simulink model "P_decouple_cascade_rov"  (Simulink 6.0)
settings: Solver=ode45  StartTime=0.0  StopTime=650  RelTol=1e-3
undefined symbols (not defined in the file): B, DQ, DQL, I, m, M, Ma, MaL, MaU, rg, sigbuilder_block, T, W, xb, xg, Xudot, yb, yg, Yvdot, zb, zg, Zwdot
libraries: simulink_extras x27, simulink x20
(part 3 of 5)

== system P_decouple_cascade_rov/outer-loop  controller/PI sine +nonlinear /Subsystem ==
  xe : Inport  Port=1  LatchInput=off
  ye : Inport  Port=2  LatchInput=off
  Divide : Product  Inputs=**/  OutScaling=2^-10
  Divide1 : Product  Inputs=**  OutScaling=2^-10
  Divide2 : Product  Inputs=***  OutScaling=2^-10
  Gain : Gain  Gain=-1
  Sine Wave : Sin  Frequency=5  Phase=pi/2  SampleTime=0
  Subtract : Sum  Inputs=+++  OutScaling=2^-10
  Subtract1 : Sum  OutScaling=2^-10
  Trigonometric Function : Trigonometry  Operator=asin
  lamda 0 : Constant  Value=0.1
  lamda 1 : Constant  Value=0.3
  lamda 2 : Constant  Value=0.5
  lamda0^2 : Math  Operator=square  SaturateOnIntegerOverflow=on
  ud : Constant  Value=0.5
  xe^2 : Math  Operator=square  SaturateOnIntegerOverflow=on
  ye^2 : Math  Operator=square  SaturateOnIntegerOverflow=on
  yaw_angle : Outport
  wires:
  lamda 0/1 -> lamda0^2/1
  lamda0^2/1 -> Subtract/1
  xe^2/1 -> Subtract/2
  ye^2/1 -> Subtract/3
  Subtract/1 -> Divide/3
  lamda 1/1 -> Divide1/1, Divide2/1
  ud/1 -> Divide1/2
  Divide1/1 -> Subtract1/1
  Divide2/1 -> Subtract1/2
  lamda 2/1 -> Divide2/2
  Sine Wave/1 -> Divide2/3
  Trigonometric Function/1 -> Gain/1
  Subtract1/1 -> Divide/1
  Divide/1 -> Trigonometric Function/1
  xe/1 -> xe^2/1
  ye/1 -> ye^2/1, Divide/2
  Gain/1 -> yaw_angle/1

== system P_decouple_cascade_rov/outer-loop  controller/outer-P decouple /inner-PI ==
  PI : Inport  Port=1  LatchInput=off
  Demux1 : Demux  Outputs=6
  Mux2 : Mux  Inputs=6
  P Controller2 : simulink_extras/Additional Linear/PID Controller  P=1  I=0  D=0
  P Controller4 : simulink_extras/Additional Linear/PID Controller  P=1  I=0  D=0
  PController1 : simulink_extras/Additional Linear/PID Controller  P=1  I=0  D=0
  PI Controller3 : simulink_extras/Additional Linear/PID Controller  P=1  I=0  D=0
  " " : Outport
  wires:
  PI Controller3/1 -> Mux2/3
  PController1/1 -> Mux2/1
  P Controller2/1 -> Mux2/2
  Demux1/1 -> PController1/1
  Demux1/2 -> P Controller2/1
  Demux1/3 -> PI Controller3/1
  Demux1/6 -> P Controller4/1
  P Controller4/1 -> Mux2/6
  PI/1 -> Demux1/1
  Mux2/1 -> " "/1

== system P_decouple_cascade_rov/outer-loop  controller/outer-sliding decouple/Subsystem ==
  xe : Inport  Port=1  LatchInput=off
  ye : Inport  Port=2  LatchInput=off
  Divide : Product  Inputs=**/  OutScaling=2^-10
  Divide1 : Product  Inputs=**  OutScaling=2^-10
  Divide2 : Product  Inputs=***  OutScaling=2^-10
  Gain : Gain  Gain=-1
  Sine Wave : Sin  Frequency=5  Phase=pi/2  SampleTime=0
  Subtract : Sum  Inputs=+++  OutScaling=2^-10
  Subtract1 : Sum  OutScaling=2^-10
  Trigonometric Function : Trigonometry  Operator=asin
  lamda 0 : Constant  Value=0.1
  lamda 1 : Constant  Value=0.3
  lamda 2 : Constant  Value=0.5
  lamda0^2 : Math  Operator=square  SaturateOnIntegerOverflow=on
  ud : Constant  Value=0.5
  xe^2 : Math  Operator=square  SaturateOnIntegerOverflow=on
  ye^2 : Math  Operator=square  SaturateOnIntegerOverflow=on
  yaw_angle : Outport
  wires:
  lamda 0/1 -> lamda0^2/1
  lamda0^2/1 -> Subtract/1
  xe^2/1 -> Subtract/2
  ye^2/1 -> Subtract/3
  Subtract/1 -> Divide/3
  lamda 1/1 -> Divide1/1, Divide2/1
  ud/1 -> Divide1/2
  Divide1/1 -> Subtract1/1
  Divide2/1 -> Subtract1/2
  lamda 2/1 -> Divide2/2
  Sine Wave/1 -> Divide2/3
  Trigonometric Function/1 -> Gain/1
  Subtract1/1 -> Divide/1
  Divide/1 -> Trigonometric Function/1
  xe/1 -> xe^2/1
  ye/1 -> ye^2/1, Divide/2
  Gain/1 -> yaw_angle/1

== system P_decouple_cascade_rov/pipeline  tracking planner  /decoupled input/x25, y=0, z=50 yaw=1.57 ==
  Mux : Mux  Inputs=6
  Start : Constant  Value=15
  Start1 : Constant  Value=25
  Start2 : Constant  Value=1.57
  6 : Outport
  wires:
  Start1/1 -> Mux/1
  Mux/1 -> 6/1
  Start2/1 -> Mux/6
  Start/1 -> Mux/3

== system P_decouple_cascade_rov/pipeline  tracking planner  /decoupled input/x=0,y=0, z=0 yaw=0   ==
  Mux : Mux  Inputs=6
  Start : Constant  Value=0
  Start1 : Constant  Value=0
  8 : Outport
  wires:
  Mux/1 -> 8/1
  Start1/1 -> Mux/1
  Start/1 -> Mux/3, Mux/2, Mux/6

== system P_decouple_cascade_rov/pipeline  tracking planner  /decoupled input/x=15,y=0, z=45 yaw=0  ==
  Mux : Mux  Inputs=6
  Start1 : Constant  Value=15
  Start2 : Constant  Value=10
  Start3 : Constant  Value=0
  Start4 : Constant  Value=0
  3 : Outport
  wires:
  Mux/1 -> 3/1
  Start1/1 -> Mux/1
  Start2/1 -> Mux/3
  Start3/1 -> Mux/6
  Start4/1 -> Mux/2

== system P_decouple_cascade_rov/pipeline  tracking planner  /decoupled input/x=25, z=45 yaw=0 ==
  Mux : Mux  Inputs=6
  Start : Constant  Value=10
  Start1 : Constant  Value=25
  Start2 : Constant  Value=0
  4 : Outport
  wires:
  Mux/1 -> 4/1
  Start1/1 -> Mux/1
  Start/1 -> Mux/3
  Start2/1 -> Mux/6

== system P_decouple_cascade_rov/pipeline  tracking planner  /decoupled input/x=25,y=0, z=50 yaw=0 ==
  Mux : Mux  Inputs=6
  Start : Constant  Value=0
  Start1 : Constant  Value=25
  Start2 : Constant  Value=15
  5 : Outport
  wires:
  Start1/1 -> Mux/1
  Mux/1 -> 5/1
  Start/1 -> Mux/6
  Start2/1 -> Mux/3

== system P_decouple_cascade_rov/pipeline  tracking planner  /decoupled input/x=25,y=40, z=50 yaw=0 ==
  Mux : Mux  Inputs=6
  Start : Constant  Value=0
  Start1 : Constant  Value=25
  Start2 : Constant  Value=15
  Start3 : Constant  Value=15
  7 : Outport
  wires:
  Start1/1 -> Mux/1
  Mux/1 -> 7/1
  Start/1 -> Mux/6
  Start2/1 -> Mux/2
  Start3/1 -> Mux/3

== system P_decouple_cascade_rov/pipeline  tracking planner  /decoupled input/x=y=0, z=-50 yaw=0   ==
  Mux : Mux  Inputs=6
  Start : Constant  Value=15
  Start1 : Constant  Value=0
  Start2 : Constant  Value=0
  "1 " : Outport
  wires:
  Mux/1 -> "1 "/1
  Start1/1 -> Mux/1, Mux/2
  Start/1 -> Mux/3
  Start2/1 -> Mux/6

== system P_decouple_cascade_rov/pipeline  tracking planner  /decoupled input/x=y=15, z=50 yaw=0  ==
  Mux : Mux  Inputs=6
  Start : Constant  Value=0
  Start1 : Constant  Value=15
  Start2 : Constant  Value=15
  2 : Outport
  wires:
  Mux/1 -> 2/1
  Start1/1 -> Mux/1
  Start2/1 -> Mux/3
  Start/1 -> Mux/6

== system P_decouple_cascade_rov/(Observer/Euler  Transformation1/Transformation matrix R/Row1 of T ==
  angular body  velocity : Inport  Port=1  LatchInput=off
  angular position : Inport  Port=2  LatchInput=off
  1 : Fcn  Expr=1
  Dot Product1 : simulink/Math Operations/Dot Product  InputSameDT=on  OutDataType=sfix(16)  OutScaling=2^-10  DoSatur=off
  Mux1 : Mux  Inputs=3
  cX.tY : Fcn  Expr=cos(u[1])*tan(u[2])
  sX.tY : Fcn  Expr=sin(u[1])*tan(u[2])
  angular earth velocity (row 1) : Outport
  wires:
  Dot Product1/1 -> angular earth velocity (row 1)/1
  angular body  velocity/1 -> Dot Product1/2
  Mux1/1 -> Dot Product1/1
  cX.tY/1 -> Mux1/3
  sX.tY/1 -> Mux1/2
  1/1 -> Mux1/1
  angular position/1 -> cX.tY/1, sX.tY/1, 1/1

== system P_decouple_cascade_rov/(Observer/Euler  Transformation1/Transformation matrix R/Row2 of T ==
  "angular body velocity " : Inport  Port=1  LatchInput=off
  angular position : Inport  Port=2  LatchInput=off
  -sX : Fcn  Expr=-sin(u[1])
  0 : Fcn  Expr=0
  Dot Product1 : simulink/Math Operations/Dot Product  InputSameDT=on  OutDataType=sfix(16)  OutScaling=2^-10  DoSatur=off
  Mux1 : Mux  Inputs=3
  cX : Fcn  Expr=cos(u[1])
  angular earth velocity (row 2) : Outport
  wires:
  Dot Product1/1 -> angular earth velocity (row 2)/1
  "angular body velocity "/1 -> Dot Product1/2
  Mux1/1 -> Dot Product1/1
  -sX/1 -> Mux1/3
  cX/1 -> Mux1/2
  0/1 -> Mux1/1
  angular position/1 -> -sX/1, cX/1, 0/1

== system P_decouple_cascade_rov/(Observer/Euler  Transformation1/Transformation matrix R/Row3 of T ==
  "angular body velocity " : Inport  Port=1  LatchInput=off
  angular position : Inport  Port=2  LatchInput=off
  1 : Fcn  Expr=0
  Dot Product1 : simulink/Math Operations/Dot Product  InputSameDT=on  OutDataType=sfix(16)  OutScaling=2^-10  DoSatur=off
  Mux1 : Mux  Inputs=3
  cX/cY : Fcn  Expr=cos(u[1])/cos(u[2])
  sX/cY : Fcn  Expr=sin(u[1])/cos(u[2])
  angular earth velocity (row 3) : Outport
  wires:
  Dot Product1/1 -> angular earth velocity (row 3)/1
  "angular body velocity "/1 -> Dot Product1/2
  Mux1/1 -> Dot Product1/1
  cX/cY/1 -> Mux1/3
  sX/cY/1 -> Mux1/2
  1/1 -> Mux1/1
  angular position/1 -> cX/cY/1, sX/cY/1, 1/1

== system P_decouple_cascade_rov/(Observer/Euler  Transformation1/Transformation matrix T/Row1 of R ==
  translational body velocity : Inport  Port=1  LatchInput=off
  angular position : Inport  Port=2  LatchInput=off
  -sZ.cX+cZ.sY.sX : Fcn  Expr=-sin(u[3])*cos(u[1]) + cos(u[3])*sin(u[2])*sin(u[1])
  Dot Product : simulink/Math Operations/Dot Product  InputSameDT=on  OutDataType=sfix(16)  OutScaling=2^-10  DoSatur=off
  Mux : Mux  Inputs=3
  cY.cZ : Fcn  Expr=cos(u[3]) * cos(u[2])
  sZ.sX+cZ.cX.sY : Fcn  Expr=sin(u[3])*sin(u[1]) + cos(u[3])*cos(u[1])*sin(u[2])
  translational earth velocity (row 1) : Outport
  wires:
  Dot Product/1 -> translational earth velocity (row 1)/1
  translational body velocity/1 -> Dot Product/2
  Mux/1 -> Dot Product/1
  sZ.sX+cZ.cX.sY/1 -> Mux/3
  -sZ.cX+cZ.sY.sX/1 -> Mux/2
  cY.cZ/1 -> Mux/1
  angular position/1 -> sZ.sX+cZ.cX.sY/1, -sZ.cX+cZ.sY.sX/1, cY.cZ/1

== system P_decouple_cascade_rov/(Observer/Euler  Transformation1/Transformation matrix T/Row2 of R ==
  translational body velocity : Inport  Port=1  LatchInput=off
  angular position : Inport  Port=2  LatchInput=off
  -cZ.sX+sY.sZ.cX : Fcn  Expr=-cos(u[3])*sin(u[1]) + sin(u[2])*sin(u[3])*cos(u[1])
  Dot Product1 : simulink/Math Operations/Dot Product  InputSameDT=on  OutDataType=sfix(16)  OutScaling=2^-10  DoSatur=off
  Mux1 : Mux  Inputs=3
  cY.sZ : Fcn  Expr=sin(u[3]) * cos(u[2])
  cZ.cX+sX.sY.sZ : Fcn  Expr=cos(u[3])*cos(u[1]) + sin(u[1])*sin(u[2])*sin(u[3])
  translational earth velocity (row 2) : Outport
  wires:
  Dot Product1/1 -> translational earth velocity (row 2)/1
  translational body velocity/1 -> Dot Product1/2
  Mux1/1 -> Dot Product1/1
  -cZ.sX+sY.sZ.cX/1 -> Mux1/3
  cZ.cX+sX.sY.sZ/1 -> Mux1/2
  cY.sZ/1 -> Mux1/1
  angular position/1 -> -cZ.sX+sY.sZ.cX/1, cZ.cX+sX.sY.sZ/1, cY.sZ/1

== system P_decouple_cascade_rov/(Observer/Euler  Transformation1/Transformation matrix T/Row3 of R ==
  translational body velocity : Inport  Port=1  LatchInput=off
  angular position : Inport  Port=2  LatchInput=off
  -sY : Fcn  Expr=-sin(u[2])
  Dot Product1 : simulink/Math Operations/Dot Product  InputSameDT=on  OutDataType=sfix(16)  OutScaling=2^-10  DoSatur=off
  Mux1 : Mux  Inputs=3
  cY.cX : Fcn  Expr=cos(u[2])*cos(u[1])
  cY.sX : Fcn  Expr=cos(u[2])*sin(u[1])
  translational earth velocity (row 3) : Outport  InitialOutput=0
  wires:
  Dot Product1/1 -> translational earth velocity (row 3)/1
  translational body velocity/1 -> Dot Product1/2
  Mux1/1 -> Dot Product1/1
  cY.cX/1 -> Mux1/3
  cY.sX/1 -> Mux1/2
  -sY/1 -> Mux1/1
  angular position/1 -> cY.cX/1, cY.sX/1, -sY/1

== system P_decouple_cascade_rov/(Observer/Thruster  Dynamic/thruster  dynamic     1/thruster  alloc.  ==
  err : Inport  Port=1  LatchInput=off
  " input" : Constant  Value=[ 1 1 1 1]'
  Selector : Selector  Elements=[1 2 3 6]  InputPortWidth=6
  thruster  allocation control1 : Subsystem  AncestorBlock=|
      | rov_design_analysis/ROV Controller
      | Design
      | Applications/1. Heading autopilot/thruster 
      | allocation control
  u : Outport
  wires:
  err/1 -> Selector/1
  Selector/1 -> thruster  allocation control1/1(vel)
  " input"/1 -> thruster  allocation control1/2(on/off)
  thruster  allocation control1/1(volt) -> u/1

== system P_decouple_cascade_rov/(Observer/inner-loop controller1/inner -PI-decouple /Centripetal & Coriolis ==
  vel : Inport  Orientation=up  Port=1  LatchInput=off
  Demux : Demux  Orientation=up  Outputs=2
  Mux : Mux  Inputs=2
  Product{1..5} (5 alike) : Product  SaturateOnIntegerOverflow=on  RndMeth=Zero  InputSameDT=on
  Rg : Constant  Value=rg
  Sum : Sum  SaturateOnIntegerOverflow=on  InputSameDT=on
  Sum1 : Sum  SaturateOnIntegerOverflow=on  InputSameDT=on
  inertia(3x3) : Gain  Gain=I  Multiplication=Matrix(K*u)  SaturateOnIntegerOverflow=on
  "mass(3x3) " : Gain  Gain=m  Multiplication=Matrix(K*u)  SaturateOnIntegerOverflow=on
  "mass(3x3)   " : Gain  Gain=m  Multiplication=Matrix(K*u)  SaturateOnIntegerOverflow=on
  force : Outport  InitialOutput=0
  wires:
  Product1/1 -> Sum/2
  "mass(3x3)   "/1 -> Product2/1
  Product2/1 -> Sum/1
  Rg/1 -> Product3/2, "mass(3x3)   "/1
  Product3/1 -> Product4/2
  Product4/1 -> Sum1/1
  Product5/1 -> Product2/2, Sum1/2
  Sum1/1 -> "mass(3x3) "/1
  Demux/2 -> Product5/1, Product3/1, Product4/1, Product1/1, inertia(3x3)/1
  Demux/1 -> Product5/2
  vel/1 -> Demux/1
  inertia(3x3)/1 -> Product1/2
  "mass(3x3) "/1 -> Mux/1
  Sum/1 -> Mux/2
  Mux/1 -> force/1

== system P_decouple_cascade_rov/(Observer/inner-loop controller1/inner -PI-decouple /Hydrodynamic  Damping ==
  vel : Inport  Port=1  LatchInput=off
  D linear : Gain  Gain=-diag(DQL)  SaturateOnIntegerOverflow=on
  damping force : Outport  InitialOutput=0
  wires:
  vel/1 -> D linear/1
  D linear/1 -> damping force/1

== system P_decouple_cascade_rov/(Observer/inner-loop controller1/inner -PI-decouple /Hydrodynamic  Damping1 ==
  vel : Inport  Port=1  LatchInput=off
  D quadratic : Gain  Gain=-diag(DQ)  SaturateOnIntegerOverflow=on
  Product : Product  SaturateOnIntegerOverflow=on  RndMeth=Zero  InputSameDT=on
  |u| : Abs  SaturateOnIntegerOverflow=on
  damping force : Outport  InitialOutput=0
  wires:
  Product/1 -> D quadratic/1
  vel/1 -> Product/1, |u|/1
  |u|/1 -> Product/2
  D quadratic/1 -> damping force/1

== system P_decouple_cascade_rov/(Observer/inner-loop controller1/inner -PI-decouple /inner-PI ==
  PI : Inport  Port=1  LatchInput=off
  Demux1 : Demux
  Ground : Ground
  Mux2 : Mux  Inputs=6
  P Controller{1..4} (4 alike) : simulink_extras/Additional Linear/PID Controller  P=1  I=0  D=0
  Selector : Selector  Elements=[1 2 3 6]  InputPortWidth=6
  " " : Outport
  wires:
  P Controller3/1 -> Mux2/3
  P Controller1/1 -> Mux2/1
  P Controller2/1 -> Mux2/2
  Selector/1 -> Demux1/1
  Demux1/1 -> P Controller1/1
  Demux1/2 -> P Controller2/1
  Demux1/3 -> P Controller3/1
  Demux1/4 -> P Controller4/1
  P Controller4/1 -> Mux2/6
  Ground/1 -> Mux2/4, Mux2/5
  PI/1 -> Selector/1
  Mux2/1 -> " "/1

== system P_decouple_cascade_rov/(Observer/inner-loop controller1/inner -PI-decouple /thruster  dynamic     1 ==
  volt : Inport  Orientation=down  Port=1  LatchInput=off
  Gain2 : Gain  Gain=0.5  SaturateOnIntegerOverflow=on
  Saturation : Saturate  UpperLimit=70  LowerLimit=-70
  "thruster  alloc. " : Subsystem
  T : Outport
  wires:
  volt/1 -> "thruster  alloc. "/1(err)
  "thruster  alloc. "/1(u) -> Gain2/1
  Saturation/1 -> T/1
  Gain2/1 -> Saturation/1

== system P_decouple_cascade_rov/(Observer/inner-loop controller1/inner -PI-decouple /upper limit (diag)    ==
  note: 7 8 9 10 11 12
  note: 1 2 3 4 5 6
  vel : Inport  Port=1  LatchInput=off
  (zg.W - zb.B)cY.sX : Fcn  Expr=-u[9]*u[3]*u[5]+u[8]*u[2]*u[6]
  (zg.W - zb.B)cY.sX1 : Fcn  Expr=u[9]*u[3]*u[4]-u[7]*u[1]*u[6]
  (zg.W - zb.B)cY.sX2 : Fcn  Expr=-u[8]*u[2]*u[4]+u[7]*u[1]*u[5]
  (zg.W - zb.B)cY.sX3 : Fcn  Expr=-u[9]*u[3]*u[2]+u[8]*u[2]*u[3]-u[12]*u[6]*u[5]+u[11]*u[5]*u[6]
  (zg.W - zb.B)cY.sX4 : Fcn  Expr=u[9]*u[3]*u[1]-u[7]*u[1]*u[3]+u[6]*u[12]*u[4]-u[4]*u[10]*u[6]
  (zg.W - zb.B)cY.sX5 : Fcn  Expr=-u[8]*u[2]*u[1]+u[7]*u[1]*u[2]-u[11]*u[5]*u[4]+u[10]*u[4]*u[5]
  Mux1 : Mux  Inputs=6
  Mux3 : Mux  Inputs=2
  Rg2 : Constant  Value="[MaU(1)  MaU(2)  MaU(3)  MaU(4)  MaU(5)  MaU(6) ]'"
  force : Outport
  wires:
  Mux1/1 -> force/1
  (zg.W - zb.B)cY.sX/1 -> Mux1/1
  (zg.W - zb.B)cY.sX1/1 -> Mux1/2
  (zg.W - zb.B)cY.sX2/1 -> Mux1/3
  (zg.W - zb.B)cY.sX3/1 -> Mux1/4
  (zg.W - zb.B)cY.sX4/1 -> Mux1/5
  (zg.W - zb.B)cY.sX5/1 -> Mux1/6
  vel/1 -> Mux3/1
  Rg2/1 -> Mux3/2
  Mux3/1 -> (zg.W - zb.B)cY.sX/1, (zg.W - zb.B)cY.sX1/1, (zg.W - zb.B)cY.sX4/1, (zg.W - zb.B)cY.sX5/1, (zg.W - zb.B)cY.sX3/1, (zg.W - zb.B)cY.sX2/1

== system P_decouple_cascade_rov/(Observer/inner-loop controller1/inner -PI-decouple /upper limit (diag)   1 ==
  note: 7 8 9 10 11 12
  note: 1 2 3 4 5 6
  vel : Inport  Port=1  LatchInput=off
  (zg.W - zb.B)cY.sX : Fcn  Expr=-u[9]*u[3]*u[5]+u[8]*u[2]*u[6]
  (zg.W - zb.B)cY.sX1 : Fcn  Expr=u[9]*u[3]*u[4]-u[7]*u[1]*u[6]
  (zg.W - zb.B)cY.sX2 : Fcn  Expr=-u[8]*u[2]*u[4]+u[7]*u[1]*u[5]
  (zg.W - zb.B)cY.sX3 : Fcn  Expr=-u[9]*u[3]*u[2]+u[8]*u[2]*u[3]-u[12]*u[6]*u[5]+u[11]*u[5]*u[6]
  (zg.W - zb.B)cY.sX4 : Fcn  Expr=u[9]*u[3]*u[1]-u[7]*u[1]*u[3]+u[6]*u[12]*u[4]-u[4]*u[10]*u[6]
  (zg.W - zb.B)cY.sX5 : Fcn  Expr=-u[8]*u[2]*u[1]+u[7]*u[1]*u[2]-u[11]*u[5]*u[4]+u[10]*u[4]*u[5]
  Mux1 : Mux  Inputs=6
  Mux3 : Mux  Inputs=2
  Rg1 : Constant  Value="[Ma(1)  Ma(2)  Ma(3)  Ma(4)  Ma(5)  Ma(6) ]'"
  force : Outport
  wires:
  Mux1/1 -> force/1
  (zg.W - zb.B)cY.sX/1 -> Mux1/1
  (zg.W - zb.B)cY.sX1/1 -> Mux1/2
  (zg.W - zb.B)cY.sX2/1 -> Mux1/3
  (zg.W - zb.B)cY.sX3/1 -> Mux1/4
  (zg.W - zb.B)cY.sX4/1 -> Mux1/5
  (zg.W - zb.B)cY.sX5/1 -> Mux1/6
  vel/1 -> Mux3/1
  Rg1/1 -> Mux3/2
  Mux3/1 -> (zg.W - zb.B)cY.sX/1, (zg.W - zb.B)cY.sX1/1, (zg.W - zb.B)cY.sX4/1, (zg.W - zb.B)cY.sX5/1, (zg.W - zb.B)cY.sX3/1, (zg.W - zb.B)cY.sX2/1

== system P_decouple_cascade_rov/(Observer/inner-loop controller1/inner -backstepping/Centripetal & Coriolis ==
  vel : Inport  Orientation=up  Port=1  LatchInput=off
  Demux : Demux  Orientation=up  Outputs=2
  Mux : Mux  Inputs=2
  Product{1..5} (5 alike) : Product  SaturateOnIntegerOverflow=on  RndMeth=Zero  InputSameDT=on
  Rg : Constant  Value=rg
  Sum : Sum  SaturateOnIntegerOverflow=on  InputSameDT=on
  Sum1 : Sum  SaturateOnIntegerOverflow=on  InputSameDT=on
  inertia(3x3) : Gain  Gain=I  Multiplication=Matrix(K*u)  SaturateOnIntegerOverflow=on
  "mass(3x3) " : Gain  Gain=m  Multiplication=Matrix(K*u)  SaturateOnIntegerOverflow=on
  "mass(3x3)   " : Gain  Gain=m  Multiplication=Matrix(K*u)  SaturateOnIntegerOverflow=on
  force : Outport  InitialOutput=0
  wires:
  Product1/1 -> Sum/2
  "mass(3x3)   "/1 -> Product2/1
  Product2/1 -> Sum/1
  Rg/1 -> Product3/2, "mass(3x3)   "/1
  Product3/1 -> Product4/2
  Product4/1 -> Sum1/1
  Product5/1 -> Product2/2, Sum1/2
  Sum1/1 -> "mass(3x3) "/1
  Demux/2 -> Product5/1, Product3/1, Product4/1, Product1/1, inertia(3x3)/1
  Demux/1 -> Product5/2
  vel/1 -> Demux/1
  inertia(3x3)/1 -> Product1/2
  "mass(3x3) "/1 -> Mux/1
  Sum/1 -> Mux/2
  Mux/1 -> force/1

== system P_decouple_cascade_rov/(Observer/inner-loop controller1/inner -backstepping/M+Ma_pert ==
  selector : Inport  Port=1  LatchInput=off
  Mux : Mux  Inputs=6
  Mux1 : Mux  Inputs=6
  Subsystem : Subsystem
  Subsystem1 : Subsystem
  Subsystem2 : Subsystem
  Subsystem3 : Subsystem
  Subsystem4 : Subsystem
  Subsystem5 : Subsystem
  M+Ma_pert : Outport
  "M " : Outport  Port=2
  wires:
  Subsystem/1(M+Ma (1,1)) -> Mux/1
  selector/1 -> Subsystem/1(M_select), Subsystem1/1(M_select), Subsystem2/1(M_select), Subsystem3/1(M_select), Subsystem4/1(M_select), Subsystem5/1(M_select)
  Subsystem1/1(M+Ma (2,2)) -> Mux/2
  Subsystem2/1(M+Ma (3,3)) -> Mux/3
  Subsystem3/1(M+Ma (4,4)) -> Mux/4
  Subsystem4/1(M+Ma (5,5)) -> Mux/5
  Subsystem5/1(M+Ma (6,6)) -> Mux/6
  Subsystem/2("M (1,1) ") -> Mux1/1
  Subsystem1/2("M (2,2) ") -> Mux1/2
  Subsystem2/2("M (3,3) ") -> Mux1/3
  Subsystem3/2("M (4,4) ") -> Mux1/4
  Subsystem4/2("M (5,5) ") -> Mux1/5
  Subsystem5/2("M (6,6) ") -> Mux1/6
  Mux/1 -> M+Ma_pert/1
  Mux1/1 -> "M "/1

== system P_decouple_cascade_rov/(Observer/inner-loop controller1/inner -backstepping/backstepping-x ==
  M+Ma_pert-x : Inport  Orientation=down  Port=1  LatchInput=off
  C+Ca+C_pert-y : Inport  Port=2  LatchInput=off
  err : Inport  Port=3  LatchInput=off
  1+(Yvdot+d_Yvdot)vr : Sum  Inputs=|++  SaturateOnIntegerOverflow=on  InputSameDT=on
  1+(Yvdot+d_Yvdot)vr1 : Sum  Inputs=|+-++  SaturateOnIntegerOverflow=on  InputSameDT=on
  Constant : Constant
  "Ku " : Constant  Value=21
  Ku1 : Gain  Gain=2
  Math Function : Math  Operator=reciprocal  SaturateOnIntegerOverflow=on
  Math Function1 : Math  Operator=square  SaturateOnIntegerOverflow=on
  Selector : Selector  Elements=[1]  InputPortWidth=6
  vp*rp2 : Product  Inputs=4  SaturateOnIntegerOverflow=on  RndMeth=Zero  InputSameDT=on
  ubar_ix : Outport
  wires:
  Constant/1 -> 1+(Yvdot+d_Yvdot)vr/1, 1+(Yvdot+d_Yvdot)vr1/4
  Math Function/1 -> vp*rp2/1
  1+(Yvdot+d_Yvdot)vr/1 -> vp*rp2/2
  1+(Yvdot+d_Yvdot)vr1/1 -> Math Function/1
  M+Ma_pert-x/1 -> vp*rp2/3, 1+(Yvdot+d_Yvdot)vr1/3
  "Ku "/1 -> Ku1/1, Math Function1/1
  Ku1/1 -> 1+(Yvdot+d_Yvdot)vr1/2
  Math Function1/1 -> 1+(Yvdot+d_Yvdot)vr1/1
  vp*rp2/1 -> ubar_ix/1
  C+Ca+C_pert-y/1 -> 1+(Yvdot+d_Yvdot)vr/2
  err/1 -> Selector/1
  Selector/1 -> vp*rp2/4

== system P_decouple_cascade_rov/(Observer/inner-loop controller1/inner -backstepping/backstepping-y ==
  M+Ma_pert-y : Inport  Orientation=down  Port=1  LatchInput=off
  m : Inport  Port=2  LatchInput=off
  "err  " : Inport  Port=3  LatchInput=off
  1+(Yvdot+d_Yvdot)vr1 : Sum  Inputs=|+-++  SaturateOnIntegerOverflow=on  InputSameDT=on
  1+mur : Sum  Inputs=|++  SaturateOnIntegerOverflow=on  InputSameDT=on
  Constant : Constant
  Demux3 : Demux  Outputs=6
  Ku1 : Gain  Gain=2
  "Kv " : Constant  Value=22
  Math Function : Math  Operator=reciprocal  SaturateOnIntegerOverflow=on
  Math Function1 : Math  Operator=square  SaturateOnIntegerOverflow=on
  vp*rp1 : Product  Inputs=3  SaturateOnIntegerOverflow=on  RndMeth=Zero  InputSameDT=on
  vp*rp2 : Product  Inputs=4  SaturateOnIntegerOverflow=on  RndMeth=Zero  InputSameDT=on
  ubar_iy : Outport
  wires:
  Constant/1 -> 1+mur/1, 1+(Yvdot+d_Yvdot)vr1/4
  Math Function/1 -> vp*rp2/1
  1+mur/1 -> vp*rp2/2
  1+(Yvdot+d_Yvdot)vr1/1 -> Math Function/1
  M+Ma_pert-y/1 -> vp*rp2/3, 1+(Yvdot+d_Yvdot)vr1/3
  "Kv "/1 -> Ku1/1, Math Function1/1
  Ku1/1 -> 1+(Yvdot+d_Yvdot)vr1/2
  Math Function1/1 -> 1+(Yvdot+d_Yvdot)vr1/1
  vp*rp2/1 -> ubar_iy/1
  vp*rp1/1 -> 1+mur/2
  m/1 -> vp*rp1/1
  Demux3/6 -> vp*rp1/3
  Demux3/2 -> vp*rp2/4
  "err  "/1 -> Demux3/1
  Demux3/1 -> vp*rp1/2

== system P_decouple_cascade_rov/(Observer/inner-loop controller1/inner -backstepping/backstepping-yaw ==
  M+Ma_pert-yaw : Inport  Orientation=down  Port=1  LatchInput=off
  C+Ca+C_pert-x : Inport  Port=2  LatchInput=off
  err : Inport  Port=3  LatchInput=off
  1+(Xudot+d_Xudot)uv : Sum  Inputs=|++  SaturateOnIntegerOverflow=on  InputSameDT=on
  1+(Yvdot+d_Yvdot)vr1 : Sum  Inputs=|+-++  SaturateOnIntegerOverflow=on  InputSameDT=on
  Constant : Constant
  "Kr " : Constant  Value=22
  Ku1 : Gain  Gain=2
  Math Function : Math  Operator=reciprocal  SaturateOnIntegerOverflow=on
  Math Function1 : Math  Operator=square  SaturateOnIntegerOverflow=on
  Selector : Selector  Elements=[6]  InputPortWidth=6
  vp*rp2 : Product  Inputs=4  SaturateOnIntegerOverflow=on  RndMeth=Zero  InputSameDT=on
  ubar_iyaw : Outport
  wires:
  Constant/1 -> 1+(Xudot+d_Xudot)uv/1, 1+(Yvdot+d_Yvdot)vr1/4
  Math Function/1 -> vp*rp2/1
  1+(Xudot+d_Xudot)uv/1 -> vp*rp2/2
  1+(Yvdot+d_Yvdot)vr1/1 -> Math Function/1
  M+Ma_pert-yaw/1 -> vp*rp2/3, 1+(Yvdot+d_Yvdot)vr1/3
  "Kr "/1 -> Ku1/1, Math Function1/1
  Ku1/1 -> 1+(Yvdot+d_Yvdot)vr1/2
  Math Function1/1 -> 1+(Yvdot+d_Yvdot)vr1/1
  vp*rp2/1 -> ubar_iyaw/1
  C+Ca+C_pert-x/1 -> 1+(Xudot+d_Xudot)uv/2
  err/1 -> Selector/1
  Selector/1 -> vp*rp2/4

== system P_decouple_cascade_rov/(Observer/inner-loop controller1/inner -backstepping/backstepping-z ==
  M+Ma_pert-z : Inport  Orientation=down  Port=1  LatchInput=off
  "err  " : Inport  Port=2  LatchInput=off
  1+(Yvdot+d_Yvdot)vr1 : Sum  Inputs=|+-++  SaturateOnIntegerOverflow=on  InputSameDT=on
  Constant : Constant
  Ku1 : Gain  Gain=2
  "Kw " : Constant  Value=23
  Math Function : Math  Operator=reciprocal  SaturateOnIntegerOverflow=on
  Math Function1 : Math  Operator=square  SaturateOnIntegerOverflow=on
  Selector : Selector  Elements=[3]  InputPortWidth=6
  vp*rp2 : Product  Inputs=3  SaturateOnIntegerOverflow=on  RndMeth=Zero  InputSameDT=on
  ubar_iz : Outport
  wires:
  Constant/1 -> 1+(Yvdot+d_Yvdot)vr1/4
  Math Function/1 -> vp*rp2/1
  1+(Yvdot+d_Yvdot)vr1/1 -> Math Function/1
  M+Ma_pert-z/1 -> 1+(Yvdot+d_Yvdot)vr1/3, vp*rp2/2
  "Kw "/1 -> Ku1/1, Math Function1/1
  Ku1/1 -> 1+(Yvdot+d_Yvdot)vr1/2
  Math Function1/1 -> 1+(Yvdot+d_Yvdot)vr1/1
  vp*rp2/1 -> ubar_iz/1
  "err  "/1 -> Selector/1
  Selector/1 -> vp*rp2/3

== system P_decouple_cascade_rov/(Observer/inner-loop controller1/inner -backstepping/thruster  dynamic     1 ==
  volt : Inport  Orientation=down  Port=1  LatchInput=off
  Gain2 : Gain  Gain=0.5  SaturateOnIntegerOverflow=on
  Saturation : Saturate  UpperLimit=70  LowerLimit=-70
  "thruster  alloc. " : Subsystem
  T : Outport
  wires:
  volt/1 -> "thruster  alloc. "/1(err)
  "thruster  alloc. "/1(u) -> Gain2/1
  Saturation/1 -> T/1
  Gain2/1 -> Saturation/1

== system P_decouple_cascade_rov/(Observer/inner-loop controller1/inner -backstepping/upper limit (diag)    ==
  note: 7 8 9 10 11 12
  note: 1 2 3 4 5 6
  vel : Inport  Port=1  LatchInput=off
  (zg.W - zb.B)cY.sX : Fcn  Expr=-u[9]*u[3]*u[5]+u[8]*u[2]*u[6]
  (zg.W - zb.B)cY.sX1 : Fcn  Expr=u[9]*u[3]*u[4]-u[7]*u[1]*u[6]
  (zg.W - zb.B)cY.sX2 : Fcn  Expr=-u[8]*u[2]*u[4]+u[7]*u[1]*u[5]
  (zg.W - zb.B)cY.sX3 : Fcn  Expr=-u[9]*u[3]*u[2]+u[8]*u[2]*u[3]-u[12]*u[6]*u[5]+u[11]*u[5]*u[6]
  (zg.W - zb.B)cY.sX4 : Fcn  Expr=u[9]*u[3]*u[1]-u[7]*u[1]*u[3]+u[6]*u[12]*u[4]-u[4]*u[10]*u[6]
  (zg.W - zb.B)cY.sX5 : Fcn  Expr=-u[8]*u[2]*u[1]+u[7]*u[1]*u[2]-u[11]*u[5]*u[4]+u[10]*u[4]*u[5]
  Mux1 : Mux  Inputs=6
  Mux3 : Mux  Inputs=2
  Rg2 : Constant  Value="[MaU(1)  MaU(2)  MaU(3)  MaU(4)  MaU(5)  MaU(6) ]'"
  force : Outport
  wires:
  Mux1/1 -> force/1
  (zg.W - zb.B)cY.sX/1 -> Mux1/1
  (zg.W - zb.B)cY.sX1/1 -> Mux1/2
  (zg.W - zb.B)cY.sX2/1 -> Mux1/3
  (zg.W - zb.B)cY.sX3/1 -> Mux1/4
  (zg.W - zb.B)cY.sX4/1 -> Mux1/5
  (zg.W - zb.B)cY.sX5/1 -> Mux1/6
  vel/1 -> Mux3/1
  Rg2/1 -> Mux3/2
  Mux3/1 -> (zg.W - zb.B)cY.sX/1, (zg.W - zb.B)cY.sX1/1, (zg.W - zb.B)cY.sX4/1, (zg.W - zb.B)cY.sX5/1, (zg.W - zb.B)cY.sX3/1, (zg.W - zb.B)cY.sX2/1

== system P_decouple_cascade_rov/(Observer/inner-loop controller1/inner -backstepping/upper limit (diag)   1 ==
  note: 7 8 9 10 11 12
  note: 1 2 3 4 5 6
  vel : Inport  Port=1  LatchInput=off
  (zg.W - zb.B)cY.sX : Fcn  Expr=-u[9]*u[3]*u[5]+u[8]*u[2]*u[6]
  (zg.W - zb.B)cY.sX1 : Fcn  Expr=u[9]*u[3]*u[4]-u[7]*u[1]*u[6]
  (zg.W - zb.B)cY.sX2 : Fcn  Expr=-u[8]*u[2]*u[4]+u[7]*u[1]*u[5]
  (zg.W - zb.B)cY.sX3 : Fcn  Expr=-u[9]*u[3]*u[2]+u[8]*u[2]*u[3]-u[12]*u[6]*u[5]+u[11]*u[5]*u[6]
  (zg.W - zb.B)cY.sX4 : Fcn  Expr=u[9]*u[3]*u[1]-u[7]*u[1]*u[3]+u[6]*u[12]*u[4]-u[4]*u[10]*u[6]
  (zg.W - zb.B)cY.sX5 : Fcn  Expr=-u[8]*u[2]*u[1]+u[7]*u[1]*u[2]-u[11]*u[5]*u[4]+u[10]*u[4]*u[5]
  Mux1 : Mux  Inputs=6
  Mux3 : Mux  Inputs=2
  Rg1 : Constant  Value="[Ma(1)  Ma(2)  Ma(3)  Ma(4)  Ma(5)  Ma(6) ]'"
  force : Outport
  wires:
  Mux1/1 -> force/1
  (zg.W - zb.B)cY.sX/1 -> Mux1/1
  (zg.W - zb.B)cY.sX1/1 -> Mux1/2
  (zg.W - zb.B)cY.sX2/1 -> Mux1/3
  (zg.W - zb.B)cY.sX3/1 -> Mux1/4
  (zg.W - zb.B)cY.sX4/1 -> Mux1/5
  (zg.W - zb.B)cY.sX5/1 -> Mux1/6
  vel/1 -> Mux3/1
  Rg1/1 -> Mux3/2
  Mux3/1 -> (zg.W - zb.B)cY.sX/1, (zg.W - zb.B)cY.sX1/1, (zg.W - zb.B)cY.sX4/1, (zg.W - zb.B)cY.sX5/1, (zg.W - zb.B)cY.sX3/1, (zg.W - zb.B)cY.sX2/1

== system P_decouple_cascade_rov/(Observer/inner-loop controller1/inner-P/thruster  dynamic     1 ==
  volt : Inport  Orientation=down  Port=1  LatchInput=off
  Gain2 : Gain  Gain=0.5  SaturateOnIntegerOverflow=on
  Saturation : Saturate  UpperLimit=70  LowerLimit=-70
  "thruster  alloc. " : Subsystem
  T : Outport
  wires:
  volt/1 -> "thruster  alloc. "/1(err)
  "thruster  alloc. "/1(u) -> Gain2/1
  Saturation/1 -> T/1
  Gain2/1 -> Saturation/1

== system P_decouple_cascade_rov/(Observer/inner-loop controller1/inner-sliding/thruster  dynamic     1 ==
  volt : Inport  Orientation=down  Port=1  LatchInput=off
  Gain2 : Gain  Gain=0.5  SaturateOnIntegerOverflow=on
  Saturation : Saturate  UpperLimit=70  LowerLimit=-70
  "thruster  alloc. " : Subsystem
  T : Outport
  wires:
  volt/1 -> "thruster  alloc. "/1(err)
  "thruster  alloc. "/1(u) -> Gain2/1
  Saturation/1 -> T/1
  Gain2/1 -> Saturation/1

== system P_decouple_cascade_rov/Thruster  Dynamic/thruster  dynamic     1/thruster  alloc. /thruster  allocation control1 ==
  vel : Inport  Orientation=down  Port=1  LatchInput=off
  on/off : Inport  Port=2  LatchInput=off
  "thruster allocation " : Subsystem
  volt : Outport
  wires:
  vel/1 -> "thruster allocation "/1(vel)
  on/off/1 -> "thruster allocation "/2(on/off)
  "thruster allocation "/1(volt) -> volt/1

== system P_decouple_cascade_rov/inner-loop controller/inner -PI-decouple /thruster  dynamic     1/thruster  alloc.  ==
  err : Inport  Port=1  LatchInput=off
  " input" : Constant  Value=[ 1 1 1 1]'
  Selector : Selector  Elements=[1 2 3 6]  InputPortWidth=6
  thruster  allocation control1 : Subsystem  AncestorBlock=|
      | rov_design_analysis/ROV Controller
      | Design
      | Applications/1. Heading autopilot/thruster 
      | allocation control
  u : Outport
  wires:
  err/1 -> Selector/1
  Selector/1 -> thruster  allocation control1/1(vel)
  " input"/1 -> thruster  allocation control1/2(on/off)
  thruster  allocation control1/1(volt) -> u/1

== system P_decouple_cascade_rov/inner-loop controller/inner -backstepping/M+Ma_pert/Subsystem ==
  M_select : Inport  Port=1  LatchInput=off
  M : Constant  Value=M(1,1)
  M1 : Constant  Value=MaU(1,1)
  M2 : Constant  Value=MaL(1,1)
  M3 : Constant  Value=0
  Multiport Switch : MultiPortSwitch  Inputs=3
  Sum5 : Sum  Inputs=+-  SaturateOnIntegerOverflow=on  InputSameDT=on
  M+Ma (1,1) : Outport
  "M (1,1) " : Outport  Port=2
  wires:
  M3/1 -> Multiport Switch/2
  M1/1 -> Multiport Switch/3
  M2/1 -> Multiport Switch/4
  Multiport Switch/1 -> Sum5/1
  M/1 -> Sum5/2, "M (1,1) "/1
  M_select/1 -> Multiport Switch/1
  Sum5/1 -> M+Ma (1,1)/1

== system P_decouple_cascade_rov/inner-loop controller/inner -backstepping/M+Ma_pert/Subsystem1 ==
  M_select : Inport  Port=1  LatchInput=off
  M : Constant  Value=M(1,1)
  M1 : Constant  Value=MaU(1,1)
  M2 : Constant  Value=MaL(1,1)
  M3 : Constant  Value=0
  Multiport Switch : MultiPortSwitch  Inputs=3
  Sum5 : Sum  Inputs=+-  SaturateOnIntegerOverflow=on  InputSameDT=on
  M+Ma (2,2) : Outport
  "M (2,2) " : Outport  Port=2
  wires:
  M3/1 -> Multiport Switch/2
  M1/1 -> Multiport Switch/3
  M2/1 -> Multiport Switch/4
  Multiport Switch/1 -> Sum5/1
  M/1 -> Sum5/2, "M (2,2) "/1
  M_select/1 -> Multiport Switch/1
  Sum5/1 -> M+Ma (2,2)/1

== system P_decouple_cascade_rov/inner-loop controller/inner -backstepping/M+Ma_pert/Subsystem2 ==
  M_select : Inport  Port=1  LatchInput=off
  M : Constant  Value=M(1,1)
  M1 : Constant  Value=MaU(1,1)
  M2 : Constant  Value=MaL(1,1)
  M3 : Constant  Value=0
  Multiport Switch : MultiPortSwitch  Inputs=3
  Sum5 : Sum  Inputs=+-  SaturateOnIntegerOverflow=on  InputSameDT=on
  M+Ma (3,3) : Outport
  "M (3,3) " : Outport  Port=2
  wires:
  M3/1 -> Multiport Switch/2
  M1/1 -> Multiport Switch/3
  M2/1 -> Multiport Switch/4
  Multiport Switch/1 -> Sum5/1
  M/1 -> Sum5/2, "M (3,3) "/1
  M_select/1 -> Multiport Switch/1
  Sum5/1 -> M+Ma (3,3)/1

== system P_decouple_cascade_rov/inner-loop controller/inner -backstepping/M+Ma_pert/Subsystem3 ==
  M_select : Inport  Port=1  LatchInput=off
  M : Constant  Value=M(1,1)
  M1 : Constant  Value=MaU(1,1)
  M2 : Constant  Value=MaL(1,1)
  M3 : Constant  Value=0
  Multiport Switch : MultiPortSwitch  Inputs=3
  Sum5 : Sum  Inputs=+-  SaturateOnIntegerOverflow=on  InputSameDT=on
  M+Ma (4,4) : Outport
  "M (4,4) " : Outport  Port=2
  wires:
  M3/1 -> Multiport Switch/2
  M1/1 -> Multiport Switch/3
  M2/1 -> Multiport Switch/4
  Multiport Switch/1 -> Sum5/1
  M/1 -> Sum5/2, "M (4,4) "/1
  M_select/1 -> Multiport Switch/1
  Sum5/1 -> M+Ma (4,4)/1

== system P_decouple_cascade_rov/inner-loop controller/inner -backstepping/M+Ma_pert/Subsystem4 ==
  M_select : Inport  Port=1  LatchInput=off
  M : Constant  Value=M(1,1)
  M1 : Constant  Value=MaU(1,1)
  M2 : Constant  Value=MaL(1,1)
  M3 : Constant  Value=0
  Multiport Switch : MultiPortSwitch  Inputs=3
  Sum5 : Sum  Inputs=+-  SaturateOnIntegerOverflow=on  InputSameDT=on
  M+Ma (5,5) : Outport
  "M (5,5) " : Outport  Port=2
  wires:
  M3/1 -> Multiport Switch/2
  M1/1 -> Multiport Switch/3
  M2/1 -> Multiport Switch/4
  Multiport Switch/1 -> Sum5/1
  M/1 -> Sum5/2, "M (5,5) "/1
  M_select/1 -> Multiport Switch/1
  Sum5/1 -> M+Ma (5,5)/1

== system P_decouple_cascade_rov/inner-loop controller/inner -backstepping/M+Ma_pert/Subsystem5 ==
  M_select : Inport  Port=1  LatchInput=off
  M : Constant  Value=M(1,1)
  M1 : Constant  Value=MaU(1,1)
  M2 : Constant  Value=MaL(1,1)
  M3 : Constant  Value=0
  Multiport Switch : MultiPortSwitch  Inputs=3
  Sum5 : Sum  Inputs=+-  SaturateOnIntegerOverflow=on  InputSameDT=on
  M+Ma (6,6) : Outport
  "M (6,6) " : Outport  Port=2
  wires:
  M3/1 -> Multiport Switch/2
  M1/1 -> Multiport Switch/3
  M2/1 -> Multiport Switch/4
  Multiport Switch/1 -> Sum5/1
  M/1 -> Sum5/2, "M (6,6) "/1
  M_select/1 -> Multiport Switch/1
  Sum5/1 -> M+Ma (6,6)/1

== system P_decouple_cascade_rov/inner-loop controller/inner -backstepping/thruster  dynamic     1/thruster  alloc.  ==
  err : Inport  Port=1  LatchInput=off
  " input" : Constant  Value=[ 1 1 1 1]'
  Selector : Selector  Elements=[1 2 3 6]  InputPortWidth=6
  thruster  allocation control1 : Subsystem  AncestorBlock=|
      | rov_design_analysis/ROV Controller
      | Design
      | Applications/1. Heading autopilot/thruster 
      | allocation control
  u : Outport
  wires:
  err/1 -> Selector/1
  Selector/1 -> thruster  allocation control1/1(vel)
  " input"/1 -> thruster  allocation control1/2(on/off)
  thruster  allocation control1/1(volt) -> u/1

== system P_decouple_cascade_rov/inner-loop controller/inner-P/thruster  dynamic     1/thruster  alloc.  ==
  err : Inport  Port=1  LatchInput=off
  " input" : Constant  Value=[ 1 1 1 1]'
  Selector : Selector  Elements=[1 2 3 6]  InputPortWidth=6
  thruster  allocation control1 : Subsystem  AncestorBlock=|
      | rov_design_analysis/ROV Controller
      | Design
      | Applications/1. Heading autopilot/thruster 
      | allocation control
  u : Outport
  wires:
  err/1 -> Selector/1
  Selector/1 -> thruster  allocation control1/1(vel)
  " input"/1 -> thruster  allocation control1/2(on/off)
  thruster  allocation control1/1(volt) -> u/1

== system P_decouple_cascade_rov/inner-loop controller/inner-sliding/thruster  dynamic     1/thruster  alloc.  ==
  err : Inport  Port=1  LatchInput=off
  " input" : Constant  Value=[ 1 1 1 1]'
  Selector : Selector  Elements=[1 2 3 6]  InputPortWidth=6
  thruster  allocation control1 : Subsystem  AncestorBlock=|
      | rov_design_analysis/ROV Controller
      | Design
      | Applications/1. Heading autopilot/thruster 
      | allocation control
  u : Outport
  wires:
  err/1 -> Selector/1
  Selector/1 -> thruster  allocation control1/1(vel)
  " input"/1 -> thruster  allocation control1/2(on/off)
  thruster  allocation control1/1(volt) -> u/1

== system P_decouple_cascade_rov/(Observer/Thruster  Dynamic/thruster  dynamic     1/thruster  alloc. /thruster  allocation control1 ==
  vel : Inport  Orientation=down  Port=1  LatchInput=off
  on/off : Inport  Port=2  LatchInput=off
  "thruster allocation " : Subsystem
  volt : Outport
  wires:
  vel/1 -> "thruster allocation "/1(vel)
  on/off/1 -> "thruster allocation "/2(on/off)
  "thruster allocation "/1(volt) -> volt/1

== system P_decouple_cascade_rov/(Observer/inner-loop controller1/inner -PI-decouple /thruster  dynamic     1/thruster  alloc.  ==
  err : Inport  Port=1  LatchInput=off
  " input" : Constant  Value=[ 1 1 1 1]'
  Selector : Selector  Elements=[1 2 3 6]  InputPortWidth=6
  thruster  allocation control1 : Subsystem  AncestorBlock=|
      | rov_design_analysis/ROV Controller
      | Design
      | Applications/1. Heading autopilot/thruster 
      | allocation control
  u : Outport
  wires:
  err/1 -> Selector/1
  Selector/1 -> thruster  allocation control1/1(vel)
  " input"/1 -> thruster  allocation control1/2(on/off)
  thruster  allocation control1/1(volt) -> u/1

== system P_decouple_cascade_rov/(Observer/inner-loop controller1/inner -backstepping/M+Ma_pert/Subsystem ==
  M_select : Inport  Port=1  LatchInput=off
  M : Constant  Value=M(1,1)
  M1 : Constant  Value=MaU(1,1)
  M2 : Constant  Value=MaL(1,1)
  M3 : Constant  Value=0
  Multiport Switch : MultiPortSwitch  Inputs=3
  Sum5 : Sum  Inputs=+-  SaturateOnIntegerOverflow=on  InputSameDT=on
  M+Ma (1,1) : Outport
  "M (1,1) " : Outport  Port=2
  wires:
  M3/1 -> Multiport Switch/2
  M1/1 -> Multiport Switch/3
  M2/1 -> Multiport Switch/4
  Multiport Switch/1 -> Sum5/1
  M/1 -> Sum5/2, "M (1,1) "/1
  M_select/1 -> Multiport Switch/1
  Sum5/1 -> M+Ma (1,1)/1

== system P_decouple_cascade_rov/(Observer/inner-loop controller1/inner -backstepping/M+Ma_pert/Subsystem1 ==
  M_select : Inport  Port=1  LatchInput=off
  M : Constant  Value=M(1,1)
  M1 : Constant  Value=MaU(1,1)
  M2 : Constant  Value=MaL(1,1)
  M3 : Constant  Value=0
  Multiport Switch : MultiPortSwitch  Inputs=3
  Sum5 : Sum  Inputs=+-  SaturateOnIntegerOverflow=on  InputSameDT=on
  M+Ma (2,2) : Outport
  "M (2,2) " : Outport  Port=2
  wires:
  M3/1 -> Multiport Switch/2
  M1/1 -> Multiport Switch/3
  M2/1 -> Multiport Switch/4
  Multiport Switch/1 -> Sum5/1
  M/1 -> Sum5/2, "M (2,2) "/1
  M_select/1 -> Multiport Switch/1
  Sum5/1 -> M+Ma (2,2)/1

== system P_decouple_cascade_rov/(Observer/inner-loop controller1/inner -backstepping/M+Ma_pert/Subsystem2 ==
  M_select : Inport  Port=1  LatchInput=off
  M : Constant  Value=M(1,1)
  M1 : Constant  Value=MaU(1,1)
  M2 : Constant  Value=MaL(1,1)
  M3 : Constant  Value=0
  Multiport Switch : MultiPortSwitch  Inputs=3
  Sum5 : Sum  Inputs=+-  SaturateOnIntegerOverflow=on  InputSameDT=on
  M+Ma (3,3) : Outport
  "M (3,3) " : Outport  Port=2
  wires:
  M3/1 -> Multiport Switch/2
  M1/1 -> Multiport Switch/3
  M2/1 -> Multiport Switch/4
  Multiport Switch/1 -> Sum5/1
  M/1 -> Sum5/2, "M (3,3) "/1
  M_select/1 -> Multiport Switch/1
  Sum5/1 -> M+Ma (3,3)/1

== system P_decouple_cascade_rov/(Observer/inner-loop controller1/inner -backstepping/M+Ma_pert/Subsystem3 ==
  M_select : Inport  Port=1  LatchInput=off
  M : Constant  Value=M(1,1)
  M1 : Constant  Value=MaU(1,1)
  M2 : Constant  Value=MaL(1,1)
  M3 : Constant  Value=0
  Multiport Switch : MultiPortSwitch  Inputs=3
  Sum5 : Sum  Inputs=+-  SaturateOnIntegerOverflow=on  InputSameDT=on
  M+Ma (4,4) : Outport
  "M (4,4) " : Outport  Port=2
  wires:
  M3/1 -> Multiport Switch/2
  M1/1 -> Multiport Switch/3
  M2/1 -> Multiport Switch/4
  Multiport Switch/1 -> Sum5/1
  M/1 -> Sum5/2, "M (4,4) "/1
  M_select/1 -> Multiport Switch/1
  Sum5/1 -> M+Ma (4,4)/1

== system P_decouple_cascade_rov/(Observer/inner-loop controller1/inner -backstepping/M+Ma_pert/Subsystem4 ==
  M_select : Inport  Port=1  LatchInput=off
  M : Constant  Value=M(1,1)
  M1 : Constant  Value=MaU(1,1)
  M2 : Constant  Value=MaL(1,1)
  M3 : Constant  Value=0
  Multiport Switch : MultiPortSwitch  Inputs=3
  Sum5 : Sum  Inputs=+-  SaturateOnIntegerOverflow=on  InputSameDT=on
  M+Ma (5,5) : Outport
  "M (5,5) " : Outport  Port=2
  wires:
  M3/1 -> Multiport Switch/2
  M1/1 -> Multiport Switch/3
  M2/1 -> Multiport Switch/4
  Multiport Switch/1 -> Sum5/1
  M/1 -> Sum5/2, "M (5,5) "/1
  M_select/1 -> Multiport Switch/1
  Sum5/1 -> M+Ma (5,5)/1

== system P_decouple_cascade_rov/(Observer/inner-loop controller1/inner -backstepping/M+Ma_pert/Subsystem5 ==
  M_select : Inport  Port=1  LatchInput=off
  M : Constant  Value=M(1,1)
  M1 : Constant  Value=MaU(1,1)
  M2 : Constant  Value=MaL(1,1)
  M3 : Constant  Value=0
  Multiport Switch : MultiPortSwitch  Inputs=3
  Sum5 : Sum  Inputs=+-  SaturateOnIntegerOverflow=on  InputSameDT=on
  M+Ma (6,6) : Outport
  "M (6,6) " : Outport  Port=2
  wires:
  M3/1 -> Multiport Switch/2
  M1/1 -> Multiport Switch/3
  M2/1 -> Multiport Switch/4
  Multiport Switch/1 -> Sum5/1
  M/1 -> Sum5/2, "M (6,6) "/1
  M_select/1 -> Multiport Switch/1
  Sum5/1 -> M+Ma (6,6)/1

== system P_decouple_cascade_rov/(Observer/inner-loop controller1/inner -backstepping/thruster  dynamic     1/thruster  alloc.  ==
  err : Inport  Port=1  LatchInput=off
  " input" : Constant  Value=[ 1 1 1 1]'
  Selector : Selector  Elements=[1 2 3 6]  InputPortWidth=6
  thruster  allocation control1 : Subsystem  AncestorBlock=|
      | rov_design_analysis/ROV Controller
      | Design
      | Applications/1. Heading autopilot/thruster 
      | allocation control
  u : Outport
  wires:
  err/1 -> Selector/1
  Selector/1 -> thruster  allocation control1/1(vel)
  " input"/1 -> thruster  allocation control1/2(on/off)
  thruster  allocation control1/1(volt) -> u/1

== system P_decouple_cascade_rov/(Observer/inner-loop controller1/inner-P/thruster  dynamic     1/thruster  alloc.  ==
  err : Inport  Port=1  LatchInput=off
  " input" : Constant  Value=[ 1 1 1 1]'
  Selector : Selector  Elements=[1 2 3 6]  InputPortWidth=6
  thruster  allocation control1 : Subsystem  AncestorBlock=|
      | rov_design_analysis/ROV Controller
      | Design
      | Applications/1. Heading autopilot/thruster 
      | allocation control
  u : Outport
  wires:
  err/1 -> Selector/1
  Selector/1 -> thruster  allocation control1/1(vel)
  " input"/1 -> thruster  allocation control1/2(on/off)
  thruster  allocation control1/1(volt) -> u/1

== system P_decouple_cascade_rov/(Observer/inner-loop controller1/inner-sliding/thruster  dynamic     1/thruster  alloc.  ==
  err : Inport  Port=1  LatchInput=off
  " input" : Constant  Value=[ 1 1 1 1]'
  Selector : Selector  Elements=[1 2 3 6]  InputPortWidth=6
  thruster  allocation control1 : Subsystem  AncestorBlock=|
      | rov_design_analysis/ROV Controller
      | Design
      | Applications/1. Heading autopilot/thruster 
      | allocation control
  u : Outport
  wires:
  err/1 -> Selector/1
  Selector/1 -> thruster  allocation control1/1(vel)
  " input"/1 -> thruster  allocation control1/2(on/off)
  thruster  allocation control1/1(volt) -> u/1

== system P_decouple_cascade_rov/Thruster  Dynamic/thruster  dynamic     1/thruster  alloc. /thruster  allocation control1/thruster allocation  ==
  note: vel to volt
  vel : Inport  Port=1  LatchInput=off
  on/off : Inport  Port=2  LatchInput=off
  Atomic Subsystem1 : Subsystem  TreatAsAtomicUnit=on
      mask Display: disp('check x >0, send \n signal to thrusters ')
  Atomic Subsystem2 : Subsystem  TreatAsAtomicUnit=on
      mask Display: disp('check y >0, send \n signal to thrusters ')
  Atomic Subsystem3 : Subsystem  TreatAsAtomicUnit=on
      mask Display: disp('check z >0, send \n signal to thrusters ')
  Atomic Subsystem4 : Subsystem  TreatAsAtomicUnit=on
      mask Display: disp('activate T3')
  Atomic Subsystem5 : Subsystem  TreatAsAtomicUnit=on
      mask Display: disp('activate T4')
  Atomic Subsystem6 : Subsystem  TreatAsAtomicUnit=on
      mask Display: disp('activate T2')
  Atomic Subsystem7 : Subsystem  TreatAsAtomicUnit=on
      mask Display: disp('activate T1')
  Atomic Subsystem8 : Subsystem  TreatAsAtomicUnit=on
      mask Display: disp('check yaw >0, send \n signal to thrusters ')
  Demux : Demux
  Demux1 : Demux
  Gain : Gain  Gain=-1
  Gain1 : Gain  Gain=-1
  Gain2 : Gain  Gain=0
  Gain3 : Gain  Gain=0
  Mux : Mux
  volt : Outport
  wires:
  Demux/1 -> Atomic Subsystem1/1(In2)
  Demux/2 -> Atomic Subsystem2/1(In2)
  Demux/3 -> Atomic Subsystem3/1(In2)
  Atomic Subsystem7/1(Out1) -> Mux/1
  vel/1 -> Demux/1
  Demux/4 -> Atomic Subsystem8/1(In2)
  on/off/1 -> Demux1/1
  Mux/1 -> volt/1
  Atomic Subsystem6/1(Out1) -> Mux/2
  Atomic Subsystem4/1(Out1) -> Mux/3
  Atomic Subsystem5/1(Out1) -> Mux/4
  Atomic Subsystem1/1(<0) -> Atomic Subsystem7/1(1), Atomic Subsystem6/1(In1)
  Atomic Subsystem2/1(<0) -> Atomic Subsystem4/1(In1), Gain/1
  Atomic Subsystem3/1(<0) -> Atomic Subsystem4/2(In2), Atomic Subsystem5/2(In2)
  Gain/1 -> Atomic Subsystem5/1(In1)
  Atomic Subsystem8/1(<0) -> Atomic Subsystem7/2(2), Gain1/1, Gain3/1, Gain2/1
  Gain1/1 -> Atomic Subsystem6/2(In2)
  Gain2/1 -> Atomic Subsystem5/3(In3)
  Demux1/1 -> Atomic Subsystem7/Enable
  Demux1/2 -> Atomic Subsystem6/Enable
  Demux1/3 -> Atomic Subsystem4/Enable
  Demux1/4 -> Atomic Subsystem5/Enable
  Gain3/1 -> Atomic Subsystem4/3(In3)

== system P_decouple_cascade_rov/inner-loop controller/inner -PI-decouple /thruster  dynamic     1/thruster  alloc. /thruster  allocation control1 ==
  vel : Inport  Orientation=down  Port=1  LatchInput=off
  on/off : Inport  Port=2  LatchInput=off
  "thruster allocation " : Subsystem
  volt : Outport
  wires:
  vel/1 -> "thruster allocation "/1(vel)
  on/off/1 -> "thruster allocation "/2(on/off)
  "thruster allocation "/1(volt) -> volt/1

== system P_decouple_cascade_rov/inner-loop controller/inner -backstepping/thruster  dynamic     1/thruster  alloc. /thruster  allocation control1 ==
  vel : Inport  Orientation=down  Port=1  LatchInput=off
  on/off : Inport  Port=2  LatchInput=off
  "thruster allocation " : Subsystem
  volt : Outport
  wires:
  vel/1 -> "thruster allocation "/1(vel)
  on/off/1 -> "thruster allocation "/2(on/off)
  "thruster allocation "/1(volt) -> volt/1

== system P_decouple_cascade_rov/inner-loop controller/inner-P/thruster  dynamic     1/thruster  alloc. /thruster  allocation control1 ==
  vel : Inport  Orientation=down  Port=1  LatchInput=off
  on/off : Inport  Port=2  LatchInput=off
  "thruster allocation " : Subsystem
  volt : Outport
  wires:
  vel/1 -> "thruster allocation "/1(vel)
  on/off/1 -> "thruster allocation "/2(on/off)
  "thruster allocation "/1(volt) -> volt/1

== system P_decouple_cascade_rov/inner-loop controller/inner-sliding/thruster  dynamic     1/thruster  alloc. /thruster  allocation control1 ==
  vel : Inport  Orientation=down  Port=1  LatchInput=off
  on/off : Inport  Port=2  LatchInput=off
  "thruster allocation " : Subsystem
  volt : Outport
  wires:
  vel/1 -> "thruster allocation "/1(vel)
  on/off/1 -> "thruster allocation "/2(on/off)
  "thruster allocation "/1(volt) -> volt/1

== system P_decouple_cascade_rov/(Observer/Thruster  Dynamic/thruster  dynamic     1/thruster  alloc. /thruster  allocation control1/thruster allocation  ==
  note: vel to volt
  vel : Inport  Port=1  LatchInput=off
  on/off : Inport  Port=2  LatchInput=off
  Atomic Subsystem1 : Subsystem  TreatAsAtomicUnit=on
      mask Display: disp('check x >0, send \n signal to thrusters ')
  Atomic Subsystem2 : Subsystem  TreatAsAtomicUnit=on
      mask Display: disp('check y >0, send \n signal to thrusters ')
  Atomic Subsystem3 : Subsystem  TreatAsAtomicUnit=on
      mask Display: disp('check z >0, send \n signal to thrusters ')
  Atomic Subsystem4 : Subsystem  TreatAsAtomicUnit=on
      mask Display: disp('activate T3')
  Atomic Subsystem5 : Subsystem  TreatAsAtomicUnit=on
      mask Display: disp('activate T4')
  Atomic Subsystem6 : Subsystem  TreatAsAtomicUnit=on
      mask Display: disp('activate T2')
  Atomic Subsystem7 : Subsystem  TreatAsAtomicUnit=on
      mask Display: disp('activate T1')
  Atomic Subsystem8 : Subsystem  TreatAsAtomicUnit=on
      mask Display: disp('check yaw >0, send \n signal to thrusters ')
  Demux : Demux
  Demux1 : Demux
  Gain : Gain  Gain=-1
  Gain1 : Gain  Gain=-1
  Gain2 : Gain  Gain=0
  Gain3 : Gain  Gain=0
  Mux : Mux
  volt : Outport
  wires:
  Demux/1 -> Atomic Subsystem1/1(In2)
  Demux/2 -> Atomic Subsystem2/1(In2)
  Demux/3 -> Atomic Subsystem3/1(In2)
  Atomic Subsystem7/1(Out1) -> Mux/1
  vel/1 -> Demux/1
  Demux/4 -> Atomic Subsystem8/1(In2)
  on/off/1 -> Demux1/1
  Mux/1 -> volt/1
  Atomic Subsystem6/1(Out1) -> Mux/2
  Atomic Subsystem4/1(Out1) -> Mux/3
  Atomic Subsystem5/1(Out1) -> Mux/4
  Atomic Subsystem1/1(<0) -> Atomic Subsystem7/1(1), Atomic Subsystem6/1(In1)
  Atomic Subsystem2/1(<0) -> Atomic Subsystem4/1(In1), Gain/1
  Atomic Subsystem3/1(<0) -> Atomic Subsystem4/2(In2), Atomic Subsystem5/2(In2)
  Gain/1 -> Atomic Subsystem5/1(In1)
  Atomic Subsystem8/1(<0) -> Atomic Subsystem7/2(2), Gain1/1, Gain3/1, Gain2/1
  Gain1/1 -> Atomic Subsystem6/2(In2)
  Gain2/1 -> Atomic Subsystem5/3(In3)
  Demux1/1 -> Atomic Subsystem7/Enable
  Demux1/2 -> Atomic Subsystem6/Enable
  Demux1/3 -> Atomic Subsystem4/Enable
  Demux1/4 -> Atomic Subsystem5/Enable
  Gain3/1 -> Atomic Subsystem4/3(In3)

== system P_decouple_cascade_rov/(Observer/inner-loop controller1/inner -PI-decouple /thruster  dynamic     1/thruster  alloc. /thruster  allocation control1 ==
  vel : Inport  Orientation=down  Port=1  LatchInput=off
  on/off : Inport  Port=2  LatchInput=off
  "thruster allocation " : Subsystem
  volt : Outport
  wires:
  vel/1 -> "thruster allocation "/1(vel)
  on/off/1 -> "thruster allocation "/2(on/off)
  "thruster allocation "/1(volt) -> volt/1

== system P_decouple_cascade_rov/(Observer/inner-loop controller1/inner -backstepping/thruster  dynamic     1/thruster  alloc. /thruster  allocation control1 ==
  vel : Inport  Orientation=down  Port=1  LatchInput=off
  on/off : Inport  Port=2  LatchInput=off
  "thruster allocation " : Subsystem
  volt : Outport
  wires:
  vel/1 -> "thruster allocation "/1(vel)
  on/off/1 -> "thruster allocation "/2(on/off)
  "thruster allocation "/1(volt) -> volt/1
